simulink model "BPN_test"  (Simulink 7.4)
settings: Solver=FixedStepDiscrete  StartTime=0.0  StopTime=10.0  FixedStep=0.01  RelTol=1e-3
undefined symbols (not defined in the file): BPNc_v_PackVoltDrop_fatal, sigbuilder_block
settings Model: Creator=lixuying  LastModifiedBy=sunsijun
settings DataIOCC: SaveFormat=StructureWithTime
settings OptimizationCC: InlineParams=on
settings DebuggingCC: SignalResolutionControl=TryResolveAll

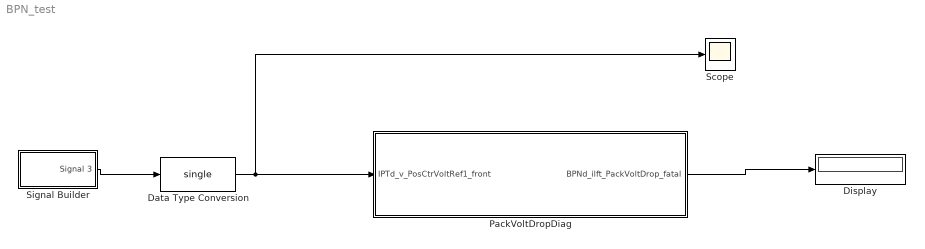
== system BPN_test ==
  Data Type Conversion : DataTypeConversion  OutDataTypeMode=single  OutDataType=fixdt(1, 16)  OutScaling=2^0  OutDataTypeStr=single
  Display : Display
  PackVoltDropDiag : Subsystem
  Scope : Scope
  Signal Builder : Subsystem  Tag=STV Subsys  LoadFcn=sigbuilder_block('load');  StartFcn=sigbuilder_block('start');  StopFcn=sigbuilder_block('stop');  ClipboardFcn=sigbuilder_block('clipboard');  mask(Sigbuilder block){}
      mask help: Sigbuilder GUI
      mask init:
      | if ~strcmp(get_param(bdroot(gcbh),'SimulationStatus'),'stopped') tuvar = sigbuilder_block('maskInit'); end
      settings: CopyFcn=sigbuilder_block('copy');  DeleteFcn=sigbuilder_block('delete');  ModelCloseFcn=sigbuilder_block('modelClose');  PreSaveFcn=sigbuilder_block('preSave');  NameChangeFcn=sigbuilder_block('namechange');  OpenFcn=sigbuilder_block('open',[437.25 199.5 550.5 399.75 ]);  CloseFcn=sigbuilder_block('close');
      mask Display: plot(0,0,100,100,[10,10,40,40,10],[80,20,20,80,80],[40,10],[50,50], [40,27,10],[65,72,56],[40,25,25,10],[28,28,43,43]);
  wires:
  Signal Builder/1(Signal 3) -> Data Type Conversion/1
  PackVoltDropDiag/1(BPNd_ilft_PackVoltDrop_fatal) -> Display/1
  Data Type Conversion/1 -> PackVoltDropDiag/1(IPTd_v_PosCtrVoltRef1_front), Scope/1

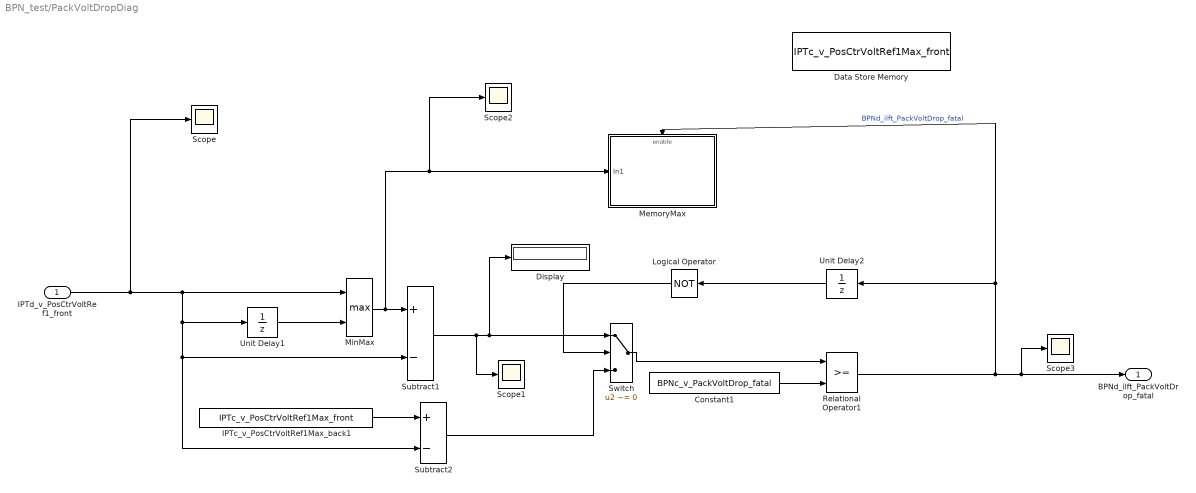
== system BPN_test/PackVoltDropDiag ==
  IPTd_v_PosCtrVoltRef1_front : Inport
  Constant1 : Constant  Value=BPNc_v_PackVoltDrop_fatal
  Data Store Memory : DataStoreMemory  DataStoreName=IPTc_v_PosCtrVoltRef1Max_front  ReadBeforeWriteMsg=warning  WriteAfterWriteMsg=warning  WriteAfterReadMsg=warning
  Display : Display
  IPTc_v_PosCtrVoltRef1Max_back1 : DataStoreRead  DataStoreName=IPTc_v_PosCtrVoltRef1Max_front  SampleTime=-1
  Logical Operator : Logic  Operator=NOT  AllPortsSameDT=off  OutDataTypeMode=boolean  OutDataTypeStr=boolean
  MemoryMax : Subsystem
  MinMax : MinMax  Function=max  Inputs=2
  Relational Operator1 : RelationalOperator  LogicOutDataTypeMode=boolean  OutDataTypeStr=boolean
  Scope{,1..3} (4 alike) : Scope
      Scope1 settings: SaveName=ScopeData2
      Scope2 settings: SaveName=ScopeData3
      Scope3 settings: SaveName=ScopeData4
  Subtract1 : Sum  Inputs=+-
  Subtract2 : Sum  Inputs=+-
  Switch : Switch  Criteria=u2 ~= 0
  Unit Delay1 : UnitDelay  SampleTime=-1
  Unit Delay2 : UnitDelay  SampleTime=-1
  BPNd_ilft_PackVoltDrop_fatal : Outport
  wires:
  Subtract1/1 -> Switch/1, Display/1, Scope1/1
  Logical Operator/1 -> Switch/2
  Unit Delay2/1 -> Logical Operator/1
  Switch/1 -> Relational Operator1/1
  MinMax/1 -> Subtract1/1, MemoryMax/1(In1), Scope2/1
  Unit Delay1/1 -> MinMax/2
  Subtract2/1 -> Switch/3
  IPTc_v_PosCtrVoltRef1Max_back1/1 -> Subtract2/1
  IPTd_v_PosCtrVoltRef1_front/1 -> MinMax/1, Subtract1/2, Subtract2/2, Unit Delay1/1, Scope/1
  Relational Operator1/1 -> MemoryMax/Enable, Unit Delay2/1, BPNd_ilft_PackVoltDrop_fatal/1, Scope3/1  "BPNd_ilft_PackVoltDrop_fatal"
  Constant1/1 -> Relational Operator1/2

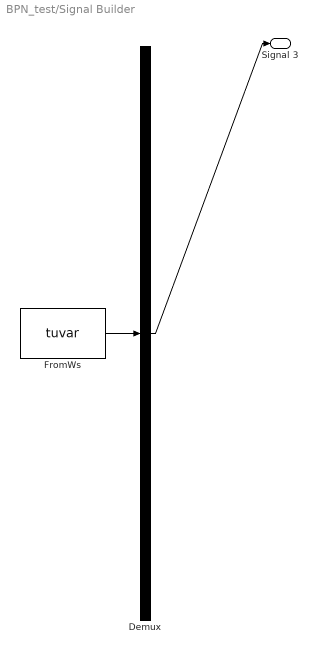
== system BPN_test/Signal Builder ==
  Demux : Demux  Tag=STV Demux  Outputs=1
  FromWs : FromWorkspace  Tag=STV FromWs  VariableName=tuvar  SampleTime=0  SigBuilderData=DataTag0  VnvData=DataTag1
      SigBuilderData=|
      | common.afterFinalStr = 'Extrapolate'
      | common.sampleTime = 0
      | dataSet.timeRange = [0 10]
      | dataSet.name = 'Group 1'
      | sbobj.Groups.Name = 'Group 1'
      | sbobj.Groups.Signals.Name = 'Signal 3'
      | sbobj.Groups.Signals.XData = [0 0.2 5 10]
      | sbobj.Groups.Signals.YData = [2000 0 1 1]
  Signal 3 : Outport  Tag=STV Outport
  wires:
  FromWs/1 -> Demux/1
  Demux/1 -> Signal 3/1

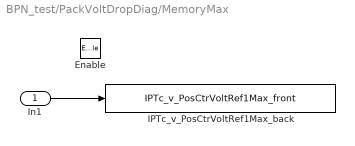
== system BPN_test/PackVoltDropDiag/MemoryMax ==
  In1 : Inport
  Enable : EnablePort
  IPTc_v_PosCtrVoltRef1Max_back : DataStoreWrite  DataStoreName=IPTc_v_PosCtrVoltRef1Max_front  SampleTime=-1
  wires:
  In1/1 -> IPTc_v_PosCtrVoltRef1Max_back/1
